simulink model "Block_LMS_uk_Ccode"  (R2017b)
settings: Solver=ode45  StartTime=0.0  StopTime=Test_time  RelTol=1e-3
values from neighbouring files (symbols this model uses):
  allFrequencyconstraints = gConstraintFun(DesignedF,Lq,plant)    [X_main_LMS.m]    (also in Z_main_LMS.m)
  eta = -50    [X_main_LMS.m]    (also in Z_main_LMS.m = -30)
  Lq = length(Qnum)    [X_main_LMS.m]    (also in Z_main_LMS.m)
  MN = minreal(plant.N * plant.M)    [X_main_LMS.m]    (also in Z_main_LMS.m)
  plant = LinearFractionalTransformation(plant)    [X_main_LMS.m]    (also in Z_main_LMS.m)
  Qnum = [7473.04093443492;-3560.91689973965;3344.74407264701;1512.08207161222;1405.87592271814;2116.43279429573;1351.87854986277;1379.05991114751;314.771935700433;497.292290224317;-533.575868853380;345.335872655316;-3440.74107426101;1735.76314107882;-4242.63151155773].'    [X_main_LMS.m]    (also in Z_main_LMS.m = [4670.29807752366;-2915.06315138601;2492.97016243023;-736.55)
undefined symbols (not defined in the file or in its folder): Ts, Vmax
settings Model: Creator=LAB_JHU  LastModifiedBy=LAB_JHU
settings DataIOCC: LimitDataPoints=on  SaveFormat=Array  SignalLoggingSaveFormat=ModelDataLogs
settings OptimizationCC: BlockReduction=off  BooleanDataType=off  LifeSpan=inf
settings DebuggingCC: SaveWithParameterizedLinksMsg=none  UnderspecifiedInitializationDetection=Classic  MergeDetectMultiDrivingBlocksExec=none  SignalResolutionControl=TryResolveAllWithWarning  MultiTaskDSMMsg=warning  MultiTaskCondExecSysMsg=none  StateNameClashWarn=warning  StrictBusMsg=None  SFUnexpectedBacktrackingDiag=warning  SFNoUnconditionalDefaultTransitionDiag=warning  SFExecutionAtInitializationDiag=none
settings HardwareCC: ProdBitPerPointer=32  ProdBitPerSizeT=32  ProdBitPerPtrDiffT=32  ProdLargestAtomicFloat=None  ProdIntDivRoundTo=Undefined  ProdEndianess=Unspecified  ProdWordSize=32  ProdHWDeviceType=32-bit Generic  TargetUnknown=on
settings ModelReferenceCC: PropagateSignalLabelsOutOfModel=off
settings CodeAppCC: StateflowObjectComments=on
settings GRTTargetCC: TargetLangStandard=C89/C90 (ANSI)  GeneratePreprocessorConditionals=Disable all
settings ConfigComp: CovMetricSettings=dw  CovHtmlReporting=on  CovSaveCumulativeToWorkspaceVar=on  CovSaveSingleToWorkspaceVar=on  CovExternalEMLEnable=off

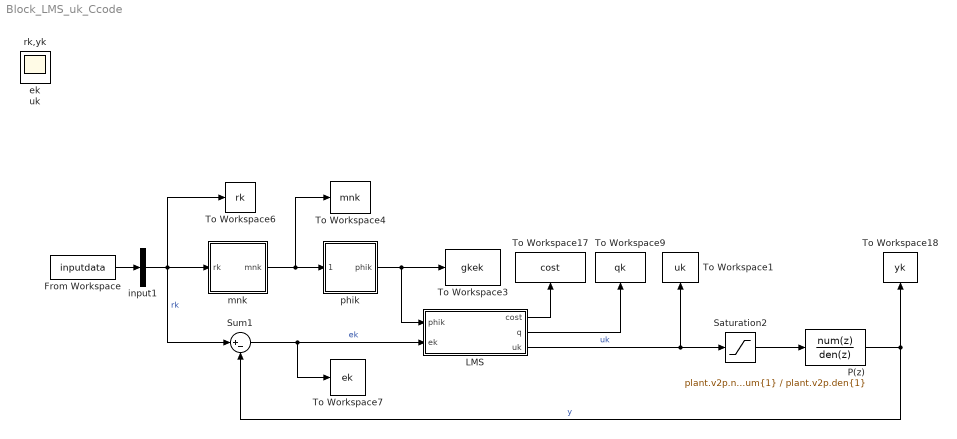
== system Block_LMS_uk_Ccode ==
  From Workspace : FromWorkspace  VariableName=inputdata  SampleTime=Ts
  LMS : Subsystem
  P(z) : DiscreteTransferFcn  Numerator=plant.v2p.num{1}  Denominator=plant.v2p.den{1}  SampleTime=0.001
  Saturation2 : Saturate  UpperLimit=Vmax  LowerLimit=-Vmax
  Sum1 : Sum  Inputs=|+-
  To Workspace1 : ToWorkspace  VariableName=uk  SampleTime=-1
  To Workspace17 : ToWorkspace  VariableName=cost  SampleTime=-1
  To Workspace18 : ToWorkspace  VariableName=yk  SampleTime=-1
  To Workspace3 : ToWorkspace  VariableName=gkek  SampleTime=-1
  To Workspace4 : ToWorkspace  VariableName=mnk  SampleTime=-1
  To Workspace6 : ToWorkspace  VariableName=rk  SampleTime=-1
  To Workspace7 : ToWorkspace  VariableName=ek  SampleTime=-1
  To Workspace9 : ToWorkspace  VariableName=qk  SampleTime=-1
  input1 : Demux  Outputs=1
  mnk : Subsystem
  phik : Subsystem
  ek : Scope
  rk,yk : Scope
  uk : Scope
  wires:
  P(z)/1 -> To Workspace18/1, Sum1/2  "y"
  mnk/1(mnk) -> To Workspace4/1, phik/1(mnk)
  Saturation2/1 -> P(z)/1
  input1/1 -> To Workspace6/1, mnk/1(rk), Sum1/1  "rk"
  phik/1(phik) -> LMS/1(phik), To Workspace3/1
  LMS/3(uk) -> Saturation2/1, To Workspace1/1  "uk"
  Sum1/1 -> LMS/2(ek), To Workspace7/1  "ek"
  LMS/2(q) -> To Workspace9/1
  LMS/1(cost) -> To Workspace17/1
  From Workspace/1 -> input1/1

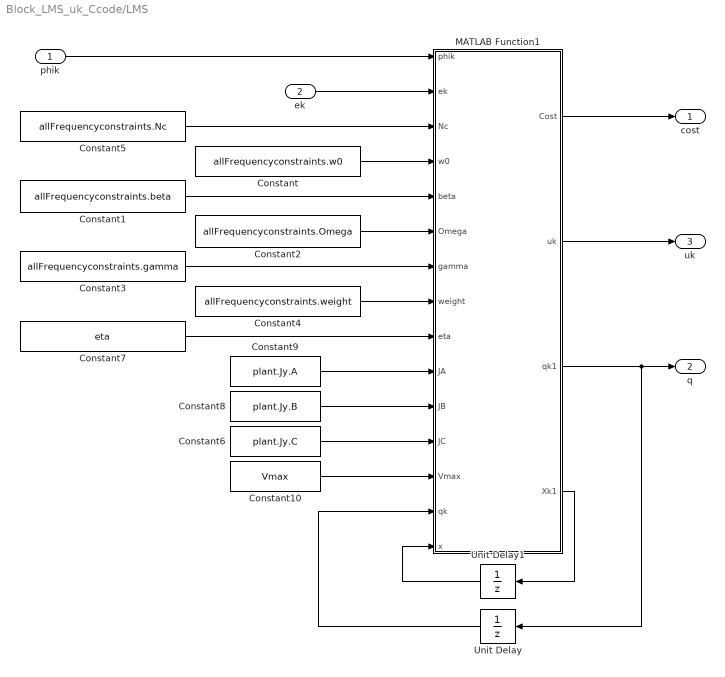
== system Block_LMS_uk_Ccode/LMS ==
  phik : Inport
  ek : Inport  Port=2
  Constant : Constant  Value=allFrequencyconstraints.w0
  Constant1 : Constant  Value=allFrequencyconstraints.beta
  Constant10 : Constant  Value=Vmax
  Constant2 : Constant  Value=allFrequencyconstraints.Omega
  Constant3 : Constant  Value=allFrequencyconstraints.gamma
  Constant4 : Constant  Value=allFrequencyconstraints.weight
  Constant5 : Constant  Value=allFrequencyconstraints.Nc
  Constant6 : Constant  Value=plant.Jy.C
  Constant7 : Constant  Value=eta
  Constant8 : Constant  Value=plant.Jy.B
  Constant9 : Constant  Value=plant.Jy.A
  MATLAB Function1 : MATLAB Function  TreatAsAtomicUnit=on
  Unit Delay : UnitDelay  InitialCondition=Qnum  SampleTime=Ts
  Unit Delay1 : UnitDelay  InitialCondition=zeros(Lq+4,1)  SampleTime=-1
  cost : Outport
  q : Outport  Port=2
  uk : Outport  Port=3
  wires:
  phik/1 -> MATLAB Function1/1(phik)
  ek/1 -> MATLAB Function1/2(ek)
  Constant5/1 -> MATLAB Function1/3(Nc)
  Constant/1 -> MATLAB Function1/4(w0)
  Constant1/1 -> MATLAB Function1/5(beta)
  Constant2/1 -> MATLAB Function1/6(Omega)
  Constant3/1 -> MATLAB Function1/7(gamma)
  Constant4/1 -> MATLAB Function1/8(weight)
  Unit Delay/1 -> MATLAB Function1/14(qk)
  Constant9/1 -> MATLAB Function1/10(JA)
  MATLAB Function1/3(qk1) -> q/1, Unit Delay/1
  MATLAB Function1/1(Cost) -> cost/1
  Constant8/1 -> MATLAB Function1/11(JB)
  Constant6/1 -> MATLAB Function1/12(JC)
  MATLAB Function1/4(Xk1) -> Unit Delay1/1
  Unit Delay1/1 -> MATLAB Function1/15(x)
  MATLAB Function1/2(uk) -> uk/1
  Constant10/1 -> MATLAB Function1/13(Vmax)
  Constant7/1 -> MATLAB Function1/9(eta)

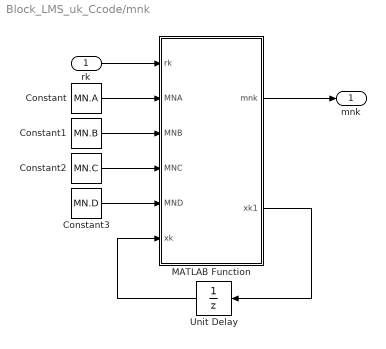
== system Block_LMS_uk_Ccode/mnk ==
  rk : Inport
  Constant : Constant  Value=MN.A
  Constant1 : Constant  Value=MN.B
  Constant2 : Constant  Value=MN.C
  Constant3 : Constant  Value=MN.D
  MATLAB Function : MATLAB Function  TreatAsAtomicUnit=on
  Unit Delay : UnitDelay  InitialCondition=zeros(length(MN.A),1)  SampleTime=-1
  mnk : Outport
  wires:
  rk/1 -> MATLAB Function/1(rk)
  MATLAB Function/1(mnk) -> mnk/1
  Constant/1 -> MATLAB Function/2(MNA)
  Constant1/1 -> MATLAB Function/3(MNB)
  Constant2/1 -> MATLAB Function/4(MNC)
  Constant3/1 -> MATLAB Function/5(MND)
  Unit Delay/1 -> MATLAB Function/6(xk)
  MATLAB Function/2(xk1) -> Unit Delay/1

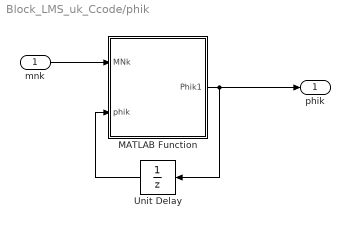
== system Block_LMS_uk_Ccode/phik ==
  mnk : Inport
  MATLAB Function : MATLAB Function  TreatAsAtomicUnit=on
  Unit Delay : UnitDelay  InitialCondition=zeros(Lq,1)  SampleTime=-1
  phik : Outport
  wires:
  MATLAB Function/1(Phik1) -> Unit Delay/1, phik/1
  mnk/1 -> MATLAB Function/1(MNk)
  Unit Delay/1 -> MATLAB Function/2(phik)

== matlab function Block_LMS_uk_Ccode/mnk/MATLAB Function ==
  data: rk input; mnk output; MNA input; MNB input; MNC input; MND input; xk input; xk1 output
function [mnk,xk1] = MNk(rk,MNA,MNB,MNC,MND,xk)

    xk1 = MNA*xk + MNB*rk;
    mnk = MNC.'*xk + MND*rk;

end

== matlab function Block_LMS_uk_Ccode/phik/MATLAB Function ==
  data: MNk input; Phik1 output; phik input
function Phik1 = Phik(MNk,phik)

    L = length(phik)-1;
    Phik1 = [MNk; reshape(phik(1:L),[L 1])];
    
end

== matlab function Block_LMS_uk_Ccode/LMS/MATLAB Function1 ==
  data: Cost output; uk output; phik input; ek input; Nc input; w0 input; beta input; Omega input; gamma input; weight input; eta input; JA input; JB input; JC input; Vmax input; qk input; qk1 output; x input; Xk1 output
function [Cost,uk,qk1,Xk1] = lms(phik,ek,Nc,w0,beta,Omega,gamma,weight,eta,JA,JB,JC,Vmax,qk,x)

fit = zeros(Nc,1); % every out of constraints
cost = w0*ek*ek/2; % function f and the min f

deltaJ = -1 * w0 * ek * phik;

for i = 1:Nc
    onebeta = beta(:,i);
    oneOmega = Omega(:,:,i);
    onegamma = gamma(i);
    oneweight = weight(i);
    g = qk.'*oneOmega*qk + onebeta.'*qk + onegamma;
    fit(i) = g;
    if g > 0
        deltaJ = deltaJ + 2*oneweight*(oneOmega*qk+onebeta);
        cost = cost + oneweight * g;
    end
end

Cost = cost;
newqk = qk + eta * deltaJ;

%% judge
q0 = newqk(1);
qxsum = newqk(2:length(newqk)).'*x(6:length(x));
E = ek;
% % general
X0 = (JA(1,:)+JB(1,2)*q0*JC(2,:))*x(1:5) + E*(JB(1,1)+JB(1,2)*q0) + JB(1,2)*qxsum;
X1 = (JA(2,:)+JB(2,2)*q0*JC(2,:))*x(1:5) + E*(JB(2,1)+JB(2,2)*q0) + JB(2,2)*qxsum;
X2 = (JA(3,:)+JB(3,2)*q0*JC(2,:))*x(1:5) + E*(JB(3,1)+JB(3,2)*q0) + JB(3,2)*qxsum;
X3 = (JA(4,:)+JB(4,2)*q0*JC(2,:))*x(1:5) + E*(JB(4,1)+JB(4,2)*q0) + JB(4,2)*qxsum;   
X4 = (JA(5,:)+JB(5,2)*q0*JC(2,:))*x(1:5) + E*(JB(5,1)+JB(5,2)*q0) + JB(5,2)*qxsum;
Z0 = E + JC(2,:)*x(1:5);
Z = x(6:length(x)-1);
Xk1 = [X0; X1; X2; X3; X4; Z0; reshape(Z,[length(Z),1])];
u = (JC(1,:)+q0*JC(2,:))*x(1:5) + E*q0 + qxsum;

if abs(u) < Vmax
    uk = u;
    qk1 = newqk;
else
    qk1 = qk;
    q0 = qk(1);
    qxsum = qk(2:length(qk)).'*x(6:length(x));
    X0 = (JA(1,:)+JB(1,2)*q0*JC(2,:))*x(1:5) + E*(JB(1,1)+JB(1,2)*q0) + JB(1,2)*qxsum;
    X1 = (JA(2,:)+JB(2,2)*q0*JC(2,:))*x(1:5) + E*(JB(2,1)+JB(2,2)*q0) + JB(2,2)*qxsum;
    X2 = (JA(3,:)+JB(3,2)*q0*JC(2,:))*x(1:5) + E*(JB(3,1)+JB(3,2)*q0) + JB(3,2)*qxsum;
    X3 = (JA(4,:)+JB(4,2)*q0*JC(2,:))*x(1:5) + E*(JB(4,1)+JB(4,2)*q0) + JB(4,2)*qxsum;   
    X4 = (JA(5,:)+JB(5,2)*q0*JC(2,:))*x(1:5) + E*(JB(5,1)+JB(5,2)*q0) + JB(5,2)*qxsum;
    Z0 = E + JC(2,:)*x(1:5);
    Z = x(6:length(x)-1);
    Xk1 = [X0; X1; X2; X3; X4; Z0; reshape(Z,[length(Z),1])];
    uk = (JC(1,:)+q0*JC(2,:))*x(1:5) + E*q0 + qxsum;
end


end
